simulink model "tcp_server"  (R2023b)
settings: Solver=FixedStepDiscrete  StartTime=0.0  StopTime=500  RelTol=1e-3
undefined symbols (not defined in the file or in its folder): Green, led0
libraries: raspberrypiBasiclib x2, raspberrypiNetworklib x1, instrumentlib x1
settings Model: Creator=seame-workstation09  LastModifiedBy=seame-workstation09
settings SolverCC: PositivePriorityOrder=on
settings OptimizationCC: EnhancedBackFolding=on  PassReuseOutputArgsAs=Individual arguments  ZeroExternalMemoryAtStartup=off  ZeroInternalMemoryAtStartup=off  MaxStackSize=64  OptimizeBlockOrder=speed  DifferentSizesBufferReuse=on  OptimizationCustomize=off  EfficientTunableParamExpr=on
settings DebuggingCC: ParameterTunabilityLossMsg=error
settings HardwareCC: ProdBitPerPointer=32  ProdBitPerSizeT=32  ProdBitPerPtrDiffT=32  ProdLargestAtomicInteger=Long  ProdLargestAtomicFloat=Double  ProdWordSize=32  ProdLongLongMode=on  ProdHWDeviceType=ARM Compatible->ARM Cortex
settings RTWCC: Description=Embedded Coder  SystemTargetFile=ert.tlc  HardwareBoard=Raspberry Pi  TLCOptions="-aInlineSetEventsForThisBaseRateFcn=TLC_FALSE -aSuppressMultiTaskScheduler=TLC_FALSE  -aRateBasedStepFcn=0"  TemplateMakefile=ert_default_tmf  Toolchain=GNU GCC Embedded Linux  BuildConfiguration=Faster Runs
settings CodeAppCC: ForceParamTrailComments=on  IgnoreCustomStorageClasses=off  OperatorAnnotations=on  SimulinkDataObjDesc=on  SFDataObjDesc=on  InsertBlockDesc=on
settings ERTTargetCC: SupportVariableSizeSignals=on  ExtModeTransport=2  ExtModeStaticAlloc=on  ExtModeMexFile=ext_xcp  ExtModeIntrfLevel=Level2 - Open

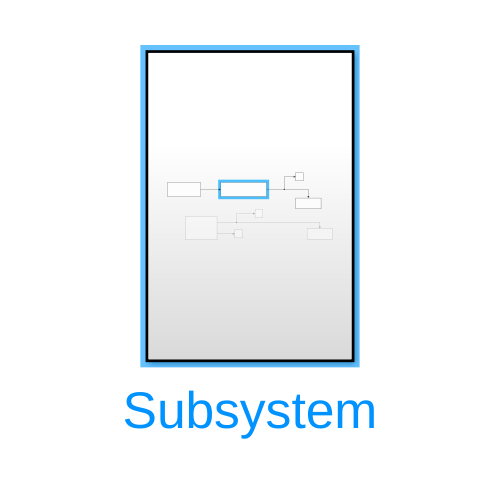
[thumbnail: Simulink's stored preview of the top-level diagram]
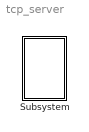
== system tcp_server ==
  Subsystem : Subsystem

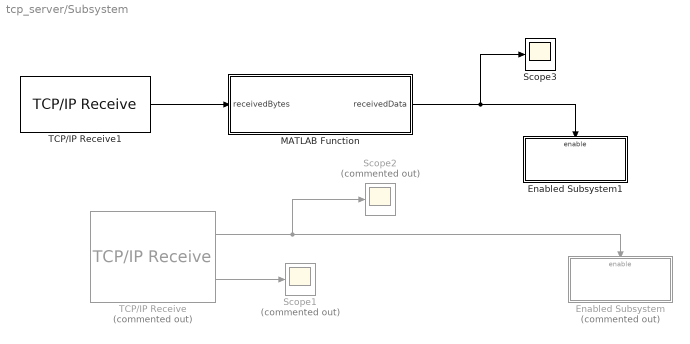
== system tcp_server/Subsystem ==
  Enabled Subsystem : Subsystem  Commented=on  TreatAsAtomicUnit=on
  Enabled Subsystem1 : Subsystem  TreatAsAtomicUnit=on
  MATLAB Function : MATLAB Function  TreatAsAtomicUnit=on
  Scope1 : Scope  Commented=on
  Scope2 : Scope  Commented=on
  Scope3 : Scope
  TCP/IP Receive : raspberrypiNetworklib/TCP//IP Receive  Commented=on  Mode_=Server  LocalServerPort_=8000  RemoteAddr_=127.0.0.1  RemoteServerPort_=25000  DataType_=uint8  DataSize_=1  SampleTime_=0.1  SimulateUsing=Code generation  ClientPortBindingSelection_=off  ClientPortToBind_=35000  BlockingMode_=off  BlockTimeout_=0.1  BlockPlatform=RASPBERRYPI
  TCP/IP Receive1 : instrumentlib/TCP//IP Receive  Host=192.168.1.154  Port=3333  DataSize=[ 1, 1 ]  DataType=uint8  ASCIIFormatting=%f  Terminator=LF  CustomTerminator=10  ByteOrder=big-endian  EnableBlockingMode=on  Timeout=10  SampleTime=0.01  SimulateUsing=Interpreted execution
  wires:
  TCP/IP Receive/2 -> Scope1/1
  TCP/IP Receive/1 -> Scope2/1, Enabled Subsystem/Enable
  TCP/IP Receive1/1 -> MATLAB Function/1(receivedBytes)
  MATLAB Function/1(receivedData) -> Scope3/1, Enabled Subsystem1/Enable

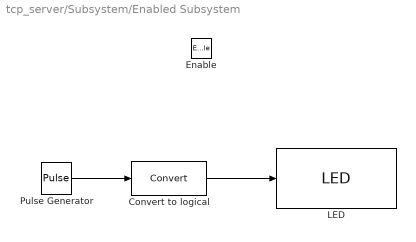
== system tcp_server/Subsystem/Enabled Subsystem ==
  Enable : EnablePort
  Convert to logical : DataTypeConversion  SaturateOnIntegerOverflow=off  RndMeth=Floor
  LED : raspberrypiBasiclib/LED  BoardProperty=Model B Rev2  LED_=led0 (Green)
  Pulse Generator : DiscretePulseGenerator  Period=10  PulseWidth=5  SampleTime=0.1
  wires:
  Convert to logical/1 -> LED/1
  Pulse Generator/1 -> Convert to logical/1

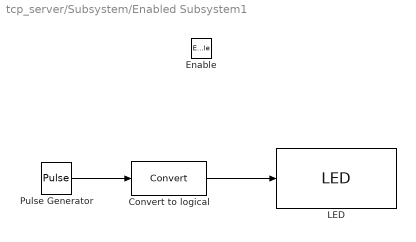
== system tcp_server/Subsystem/Enabled Subsystem1 ==
  Enable : EnablePort
  Convert to logical : DataTypeConversion  SaturateOnIntegerOverflow=off  RndMeth=Floor
  LED : raspberrypiBasiclib/LED  BoardProperty=Model B Rev2  LED_=led0 (Green)
  Pulse Generator : DiscretePulseGenerator  Period=10  PulseWidth=5  SampleTime=0.1
  wires:
  Convert to logical/1 -> LED/1
  Pulse Generator/1 -> Convert to logical/1

== matlab function tcp_server/Subsystem/MATLAB Function ==
  data: receivedBytes input; receivedData output
% Simulink에서 받은 uint8 데이터를 int32로 변환하는 함수
function receivedData = unpackData(receivedBytes)
    % 받은 바이트 배열의 길이가 4의 배수인지 확인
    if mod(length(receivedBytes), 4) ~= 0
        error('Input data length must be a multiple of 4 to convert from uint8 to int32');
    end

    % 데이터 언패킹
    receivedData = typecast(receivedBytes, 'int32');
end
